simulink model "VOO_finalversion"  (R2022a)
settings: Solver=FixedStepAuto  StartTime=0.0  StopTime=10.0  FixedStep=1e-3  RelTol=1e-3  EnableMultiTasking=on
undefined symbols (not defined in the file): D10, D11, D12, D2, D4, D5, D7, D8, D9, PTA0, PTA2, PTB23, PTB9, PTC3, PTC4, PTD0, PTD2, PTD3
libraries: frdmk64flib x10
settings Model: ExtModeTrigDuration=5  Creator=jacqu  LastModifiedBy=chris
settings OptimizationCC: EnhancedBackFolding=on  PassReuseOutputArgsAs=Individual arguments  ZeroExternalMemoryAtStartup=off  ZeroInternalMemoryAtStartup=off  MaxStackSize=64  OptimizeBlockOrder=speed  DifferentSizesBufferReuse=on  OptimizationCustomize=off  EfficientTunableParamExpr=on
settings DebuggingCC: ParameterTunabilityLossMsg=error
settings HardwareCC: ProdBitPerPointer=32  ProdBitPerSizeT=32  ProdBitPerPtrDiffT=32  ProdLargestAtomicInteger=Long  ProdLargestAtomicFloat=Double  ProdWordSize=32  ProdHWDeviceType=ARM Compatible->ARM Cortex
settings SFSimCC: MATLABDynamicMemAlloc=off
settings RTWCC: SystemTargetFile=ert.tlc  HardwareBoard=NXP FRDM-K64F  TLCOptions="-aInlineSetEventsForThisBaseRateFcn=TLC_FALSE -aSuppressMultiTaskScheduler=TLC_FALSE  -aRateBasedStepFcn=0"  TemplateMakefile=ert_default_tmf  Toolchain=GNU Tools for ARM Embedded Processors
settings CodeAppCC: ForceParamTrailComments=on  IgnoreCustomStorageClasses=off  OperatorAnnotations=on  SimulinkDataObjDesc=on  SFDataObjDesc=on  InsertBlockDesc=on
settings ERTTargetCC: ExtModeTransport=4  ExtModeMexFile=sendToCommService

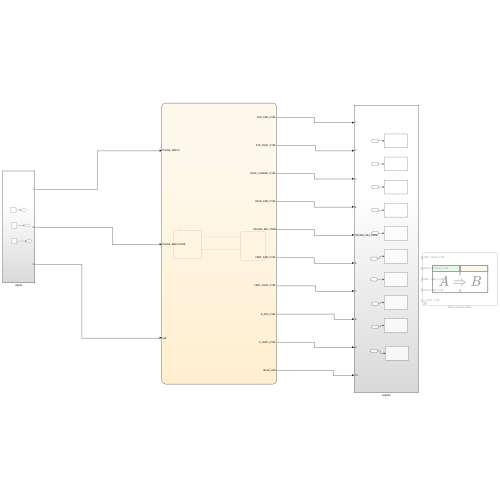
[thumbnail: Simulink's stored preview of the top-level diagram]
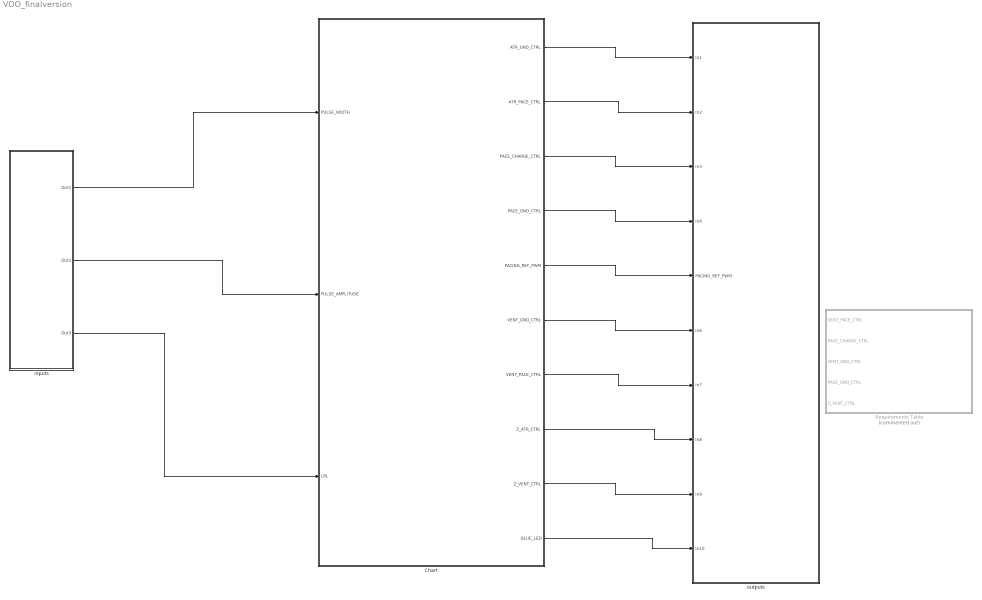
== system VOO_finalversion ==
  Chart : Stateflow chart  TreatAsAtomicUnit=on
  Requirements Table : Requirements Table  Commented=on  TreatAsAtomicUnit=on
  inputs : Subsystem
  outputs : Subsystem
  wires:
  inputs/1(Out1) -> Chart/1(PULSE_WIDTH)
  inputs/2(Out2) -> Chart/2(PULSE_AMPLITUDE)
  inputs/3(Out3) -> Chart/3(LRL)
  Chart/1(ATR_GND_CTRL) -> outputs/1(In1)
  Chart/2(ATR_PACE_CTRL) -> outputs/2(In2)
  Chart/3(PACE_CHARGE_CTRL) -> outputs/3(In3)
  Chart/4(PACE_GND_CTRL) -> outputs/4(In4)
  Chart/5(PACING_REF_PWM) -> outputs/5(PACING_REF_PWM)
  Chart/6(VENT_GND_CTRL) -> outputs/6(In6)
  Chart/7(VENT_PACE_CTRL) -> outputs/7(In7)
  Chart/8(Z_ATR_CTRL) -> outputs/8(In8)
  Chart/9(Z_VENT_CTRL) -> outputs/9(In9)
  Chart/10(BLUE_LED) -> outputs/10(In10)

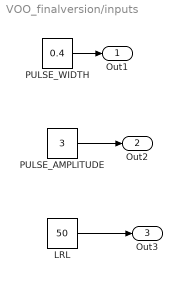
== system VOO_finalversion/inputs ==
  LRL : Constant  Value=50
  PULSE_AMPLITUDE : Constant  Value=3
  PULSE_WIDTH : Constant  Value=0.4
  Out1 : Outport
  Out2 : Outport  Port=2
  Out3 : Outport  Port=3
  wires:
  PULSE_WIDTH/1 -> Out1/1
  PULSE_AMPLITUDE/1 -> Out2/1
  LRL/1 -> Out3/1

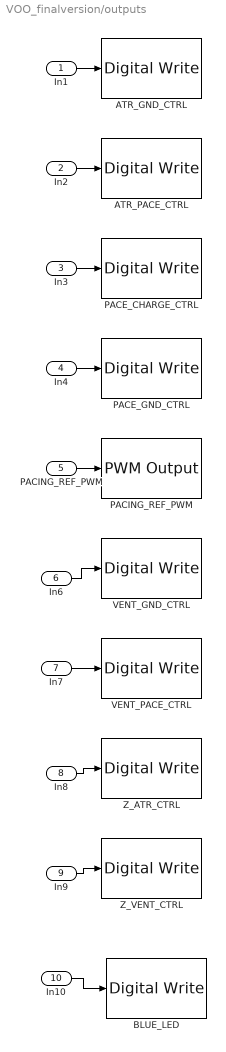
== system VOO_finalversion/outputs ==
  In1 : Inport
  In2 : Inport  Port=2
  In3 : Inport  Port=3
  In4 : Inport  Port=4
  PACING_REF_PWM : Inport  Port=5
  In6 : Inport  Port=6
  In7 : Inport  Port=7
  In8 : Inport  Port=8
  In9 : Inport  Port=9
  In10 : Inport  Port=10
  " PACING_REF_PWM" : frdmk64flib/PWM Output  Whichpin=PTA2 (D5)  InitialFrequency=2000  InitialDutyCycle=50
  ATR_GND_CTRL : frdmk64flib/Digital Write  Whichpin=PTD2 (D11)
  ATR_PACE_CTRL : frdmk64flib/Digital Write  Whichpin=PTA0 (D8)
  BLUE_LED : frdmk64flib/Digital Write  Whichpin=BLUE_LED
  PACE_CHARGE_CTRL : frdmk64flib/Digital Write  Whichpin=PTB9 (D2)
  PACE_GND_CTRL : frdmk64flib/Digital Write  Whichpin=PTD0 (D10)
  VENT_GND_CTRL : frdmk64flib/Digital Write  Whichpin=PTD3 (D12)
  VENT_PACE_CTRL : frdmk64flib/Digital Write  Whichpin=PTC4 (D9)
  Z_ATR_CTRL : frdmk64flib/Digital Write  Whichpin=PTB23 (D4)
  Z_VENT_CTRL : frdmk64flib/Digital Write  Whichpin=PTC3 (D7)
  wires:
  In1/1 -> ATR_GND_CTRL/1
  In2/1 -> ATR_PACE_CTRL/1
  In3/1 -> PACE_CHARGE_CTRL/1
  In4/1 -> PACE_GND_CTRL/1
  PACING_REF_PWM/1 -> " PACING_REF_PWM"/1
  In6/1 -> VENT_GND_CTRL/1
  In7/1 -> VENT_PACE_CTRL/1
  In8/1 -> Z_ATR_CTRL/1
  In9/1 -> Z_VENT_CTRL/1
  In10/1 -> BLUE_LED/1

== stateflow chart VOO_finalversion/Requirements Table ==
  (default) -> (junction 1073742649)
  (junction 1073742649) -> (junction 1073742650) : {
      | % SF_REQ_REV_07
      | }
  (junction 1073742650) -> (junction 1073742652) : {
      | % HEADER_ASSIGNMENTS
      |
      | }
  (junction 1073742652) -> (junction 1073742654) : {
      | % START_A_4
      | }
  (junction 1073742654) -> (junction 1073742656) : {
      | }
  (junction 1073742656) -> (junction 1073742658)
  (junction 1073742658) -> (junction 1073742660) : {
      | }
  (junction 1073742660) -> (junction 1073742662) : {
      | % END_A_4
      | }
  (junction 1073742662) -> (junction 1073742664) : {
      | % START_R_1
      | }
  (junction 1073742664) -> (junction 1073742666) : {
      | }
  (junction 1073742666) -> (junction 1073742668) : {
      |
      |
      | }
  (junction 1073742668) -> (junction 1073742670) : {
      | }
  (junction 1073742670) -> (junction 1073742672) : {
      | % START_R_10
      | }
  (junction 1073742672) -> (junction 1073742674) : {
      | }
  (junction 1073742674) -> (junction 1073742676)
  (junction 1073742676) -> (junction 1073742678) [order 1] : [duration((prev(VENT_PACE_CTRL)==false) && (prev(PACE_CHARGE_CTRL) == true) && (prev(VENT_GND_CTRL)==true) && (prev(PACE_GND_CTRL)==true) && (prev(Z_VENT_CTRL)==false)) >= ((60000/LRL)-PULSE_WIDTH)/1000]
  (junction 1073742676) -> (junction 1073742684) [order 2]
  (junction 1073742678) -> (junction 1073742680) : {
      | reqtable_postcondition((VENT_PACE_CTRL == true) && (PACE_CHARGE_CTRL == false) && (VENT_GND_CTRL == false) && (PACE_GND_CTRL == true) && (Z_VENT_CTRL == false), 'R:1.1');
      |
      |
      | }
  (junction 1073742680) -> (junction 1073742682) : {
      | }
  (junction 1073742682) -> (junction 1073742684)
  (junction 1073742684) -> (junction 1073742686)
  (junction 1073742686) -> (junction 1073742688) : {
      | % END_R_10
      | }
  (junction 1073742688) -> (junction 1073742690) : {
      | % START_R_16
      | }
  (junction 1073742690) -> (junction 1073742692) : {
      | }
  (junction 1073742692) -> (junction 1073742694)
  (junction 1073742694) -> (junction 1073742696) [order 1] : [duration((prev(VENT_PACE_CTRL)==true) && (prev(PACE_CHARGE_CTRL) == false) && (prev(VENT_GND_CTRL)==false) && (prev(PACE_GND_CTRL)==true) && (prev(Z_VENT_CTRL)==false)) >= (PULSE_WIDTH)/1000]
  (junction 1073742694) -> (junction 1073742702) [order 2]
  (junction 1073742696) -> (junction 1073742698) : {
      | reqtable_postcondition((VENT_PACE_CTRL == false) && (PACE_CHARGE_CTRL == true) && (VENT_GND_CTRL == true) && (PACE_GND_CTRL == true) && (Z_VENT_CTRL == false), 'R:1.2');
      |
      |
      | }
  (junction 1073742698) -> (junction 1073742700) : {
      | }
  (junction 1073742700) -> (junction 1073742702)
  (junction 1073742702) -> (junction 1073742704)
  (junction 1073742704) -> (junction 1073742706) : {
      | % END_R_16
      | }
  (junction 1073742706) -> (junction 1073742708) : {
      | % END_R_1
      | }
  data: VENT_PACE_CTRL input boolean; PACE_CHARGE_CTRL input boolean; VENT_GND_CTRL input boolean; PACE_GND_CTRL input boolean; Z_VENT_CTRL input boolean; PULSE_WIDTH constant double; HEART_RATE constant double

== stateflow chart VOO_finalversion/Chart ==
  state PACE_OFF
    entry:
    ATR_PACE_CTRL = 0
    VENT_PACE_CTRL = 0
    PACING_REF_PWM = 20*PULSE_AMPLITUDE
    PACE_CHARGE_CTRL = 1
    PACE_GND_CTRL = 1
    VENT_PACE_CTRL = 0
    Z_ATR_CTRL = 0
    Z_VENT_CTRL = 0
    ATR_PACE_CTRL = 0
    ATR_GND_CTRL = 0
    VENT_GND_CTRL = 1
    BLUE_LED = 0
  state PACE_ON
    entry:
    PACE_CHARGE_CTRL = 0
    PACE_GND_CTRL = 1
    ATR_PACE_CTRL = 0
    ATR_GND_CTRL = 0
    Z_ATR_CTRL = 0
    Z_VENT_CTRL = 0
    VENT_GND_CTRL = 0
    VENT_PACE_CTRL = 1
    BLUE_LED = 1
  note: at paceoff state, waiting for pacing on.
  note: after period-pulsewidth, paceoff turns into pace on. it paced for a pulse width and go back to pace_off again.
  (default) -> PACE_OFF
  PACE_OFF -> PACE_ON : [after((60000/LRL)-PULSE_WIDTH,msec)]
  PACE_ON -> PACE_OFF : [after(PULSE_WIDTH,msec)]
  data: PULSE_WIDTH input; PULSE_AMPLITUDE input; ATR_GND_CTRL output; ATR_PACE_CTRL output; PACE_CHARGE_CTRL output; PACE_GND_CTRL output; PACING_REF_PWM output; VENT_GND_CTRL output; VENT_PACE_CTRL output; Z_ATR_CTRL output; Z_VENT_CTRL output; BLUE_LED output; LRL input
